simulink model "MSDRPrimaryLoop_LoadFollow"  (R2021b)
settings: Solver=VariableStepAuto  StartTime=0.0  StopTime=604900  MaxStep=1  MinStep=0.01  RelTol=1e-3
undefined symbols (not defined in the file): a_f, A_free_PHX, a_g, A_h_PHX, beta, beta_t, bubbleGeneratorArea, bubbleGeneratorDh, bubbleGeneratorElevation, bubbleGeneratorLength, bubbleGeneratorVolume, bubbleSaturationLevel, bubbleSeparatorArea, bubbleSeparatorDiameter, bubbleSeparatorDo, bubbleSeparatorLength, bubbleSeparatorSlope, bypassRatio, C0, coreFlowArea, coreFuelVolume, coreLowerPlenumArea, coreLowerPlenumHydraulicDiameter, coreLowerPlenumLength, coreLowerPlenumVolume, coreUpperPlenumArea, coreUpperPlenumHydraulicDiameter, coreUpperPlenumLength, coreUpperPlenumVolume, coreVolume, cpGraphite, dissolusionRatio, dMin, dScale, dsmConst, DXeG, Fiss_factor, fuelChannelHydrualicDiameter, fuelChannelLength, fuelDepositRatio, fuelFraction, fuelGraphiteArea, fuelGraphiteHeatTransferCoefficient, gamma0, gamma1, gamma2, generatorDsm, graphiteKDiff, graphiteUnitCellThickness, initialIodineConcentration, InitialXeMolarConcentration, InjectionRatio, injectionRatio, iodineDecayConstant, IodineDecayConstant, iodineYield, kGraphite, kScale, Lam, lam ... (+60)
libraries: fl_lib x268, nesl_utility x106, SimscapeFluids_lib x20, slpidlib x1
(part 10 of 12)

== system MSDRPrimaryLoop_LoadFollow/Chemical Processing/PipeLine/XenonCalc/InterphaseTranfser/Constitutive ==
  alpha : Inport
  PLoss : Inport  Port=2
  VolumeRate : Inport  Port=3
  Diam : Inport  Port=4
  Absolute Reference (TL) : fl_lib/Thermal Liquid/Elements/Absolute Reference (TL)
      settings: SourceProductBaseCode=SS
  DiffusivityScale : Subsystem  ReferencedSubsystem=DiffusivityScale
  Divide : Product  Inputs=**/
  Divide1 : Product  Inputs=*/
  KScale : Subsystem  ReferencedSubsystem=KScale
  PS-Simulink Converter : nesl_utility/PS-Simulink Converter  PhysicalDomain=network_engine_domain  SubClassName=ps_output  LeftPortType=input  RightPortType=output  PseudoPeriodic=off  Frequencies=[]  Unit=inherit  AffineConversion=off
      settings: SourceProductBaseCode=PW,SS
  PS-Simulink Converter2 : nesl_utility/PS-Simulink Converter  PhysicalDomain=network_engine_domain  SubClassName=ps_output  LeftPortType=input  RightPortType=output  PseudoPeriodic=off  Frequencies=[]  Unit=inherit  AffineConversion=off
      settings: SourceProductBaseCode=PW,SS
  Pressure & Temperature Sensor (TL) : fl_lib/Thermal Liquid/Sensors/Pressure & Temperature Sensor (TL)
      settings: SourceProductBaseCode=SS  InternalSimscapePortConfiguration="{\"Bottom\":[],\"Left\":[{\"id\":\"A\",\"label\":\"A\",\"type\":\"foundation.thermal_liquid.thermal_liquid\"}],\"Right\":[{\"id\":\"B\",\"label\":\"B\",\"type\":\"foundation.thermal_liquid.thermal_liquid\"},{\"id\":\"P\",\"label\":\"P\",\"type\":\"output\"},{\"id\":\"T\",\"label\":\"T\",\"type\":\"output\"}],\"Top\":[]}"
  RateToVelocity : Gain  Gain=1/Area
  Simscape Component : SimscapeComponentBlock  SourceFile=TL_FullSensor  ComponentPath=TL_FullSensor  ComponentVariants="[\"TL_FullSensor\"]"  ComponentVariantNames="[\"TL_FullSensor\"]"  ClassName=TL_FullSensor  SchemaVersion=1
      settings: CopyFcn=simscape.engine.sli.internal.componentblockcallback(gcbh,'COPY')  PreCopyFcn=simscape.engine.sli.internal.componentblockcallback(gcbh,'PRECOPY')  PreDeleteFcn=simscape.engine.sli.internal.componentblockcallback(gcbh,'PREDELETE')  InternalSimscapePortConfiguration="{\"Bottom\":[],\"Left\":[{\"id\":\"A\",\"label\":\"A\",\"type\":\"foundation.thermal_liquid.thermal_liquid\"}],\"Right\":[{\"id\":\"U\",\"label\":\"u\",\"type\":\"output\"},{\"id\":\"RHO\",\"label\":\"rho\",\"type\":\"output\"},{\"id\":\"CP\",\"label\":\"cp\",\"type\":\"output\"},{\"id\":\"NU\",\"label\":\"nu\",\"type\":\"output\"}],\"Top\":[]}"
      mask Type: Thermodynamic Properties Sensor (TL)
  Subsystem : Subsystem
      settings: PortSchema="{\"entries\":[{\"content\":{\"sides\":[{\"content\":{\"connectorIds\":[\"In1\",\"In2\",\"In3\"]},\"type\":\"ConnectorPlacement.EquallySpacedRectSide\",\"uuid\":\"dd1c86c2-327e-41b5-90e0-a07cc4f7a239\"},{\"content\":{\"connectorIds\":[\"Out1\",\"Out2\"],\"side\":\"RIGHT\"},\"type\":\"ConnectorPlacement.EquallySpacedRectSide\",\"uuid\":\"1daff71e-8b5d-4f35-9ce7-352085350762\"},{\"content\":{\"connectorIds\":[],\"side\":\"TOP\"},\"type\":\"ConnectorPlacement.EquallySpacedRectSide\",\"uuid\":\"6cf7e847-c1ca-4561-96b9-90e4339d236b\"},{\"content\":{\"connectorIds\":[\"RConn1\"],\"side\":\"BOTTOM\"},\"type\":\"ConnectorPlacement.EquallySpacedRectSide\",\"uuid\":\"444ecab7-0e05-438f-8395-0556f9cb1910\"}]},\"type\":\"ConnectorPlacement.EquallySpacedConnector\",\"uuid\":\"a820de5e-57ef-4a78-919f-756fbb4a48db\"}],\"packageUris\":[\"http://schema.mathworks.com/mf0/Connector/R2020b\"],\"version\":\"1.0\"}"
  Ref : PMIOPort  Side=Left
  ul : Outport
  ug : Outport  Port=2
  K : Outport  Port=3
  Re : Outport  Port=4
  Sc : Outport  Port=5
  Diff : Outport  Port=6
  alphaC : Outport  Port=7
  dsm : Outport  Port=8
  f_m : Outport  Port=9
  wires:
  alpha/1 -> alphaC/1
  VolumeRate/1 -> RateToVelocity/1
  RateToVelocity/1 -> ug/1, Subsystem/3(ul), ul/1, Divide/1
  Diam/1 -> Subsystem/2(Dh), Divide/2
  PS-Simulink Converter/1 -> Divide/3, Divide1/1
  PS-Simulink Converter2/1 -> DiffusivityScale/1, KScale/1
  DiffusivityScale/1 -> Divide1/2, Diff/1
  Divide1/1 -> Sc/1
  KScale/1 -> K/1
  Subsystem/2(dsm) -> dsm/1
  Divide/1 -> Re/1
  Subsystem/1(f_Combined) -> f_m/1
  PLoss/1 -> Subsystem/1(PLoss)
  connections:
  Pressure & Temperature Sensor (TL)/LConn1 -- Simscape Component/LConn1 -- Ref/RConn1 -- Subsystem/RConn1
  Simscape Component/RConn4 -- PS-Simulink Converter/LConn1
  Pressure & Temperature Sensor (TL)/RConn3 -- PS-Simulink Converter2/LConn1
  Pressure & Temperature Sensor (TL)/RConn1 -- Absolute Reference (TL)/LConn1

== system MSDRPrimaryLoop_LoadFollow/Chemical Processing/PipeLine/XenonCalc/Salt/InPipeGeneration ==
  IodineSNumberDensity : Inport
  T_f_ave : Inport  Port=2
  DecayXenonGenerationRate : Product
  Molar/s : Product  Inputs=*/
  Na : Constant  Value=6.022e23
  T2Rho : Fcn  Expr=3960 - 0.6724*u
  gain : Gain  Gain=iodineDecayConstant*Volume
  kg/s : Gain  Gain=0.135
  "XenonGenerationRate, [kg/s]" : Outport
  wires:
  IodineSNumberDensity/1 -> gain/1
  T_f_ave/1 -> T2Rho/1
  gain/1 -> DecayXenonGenerationRate/1
  T2Rho/1 -> DecayXenonGenerationRate/2
  DecayXenonGenerationRate/1 -> Molar/s/1
  Na/1 -> Molar/s/2
  Molar/s/1 -> kg/s/1
  kg/s/1 -> "XenonGenerationRate, [kg/s]"/1

== system MSDRPrimaryLoop_LoadFollow/Chemical Processing/PipeLine/XenonCalc/Salt/Subsystem1 ==
  Gas : Inport
  Add1 : Sum  Inputs=+-
  Constant : Constant
  Subsystem : Subsystem  ReferencedSubsystem=GasToAlpha
  1-alpha : Outport
  wires:
  Gas/1 -> Subsystem/1
  Constant/1 -> Add1/1
  Subsystem/1 -> Add1/2
  Add1/1 -> 1-alpha/1

== system MSDRPrimaryLoop_LoadFollow/PHX/PHX Ideal/XenonCalc/InterphaseTranfser/Constitutive ==
  alpha : Inport
  PLoss : Inport  Port=2
  VolumeRate : Inport  Port=3
  Diam : Inport  Port=4
  Absolute Reference (TL) : fl_lib/Thermal Liquid/Elements/Absolute Reference (TL)
      settings: SourceProductBaseCode=SS
  DiffusivityScale : Subsystem  ReferencedSubsystem=DiffusivityScale
  Divide : Product  Inputs=**/
  Divide1 : Product  Inputs=*/
  KScale : Subsystem  ReferencedSubsystem=KScale
  PS-Simulink Converter : nesl_utility/PS-Simulink Converter  PhysicalDomain=network_engine_domain  SubClassName=ps_output  LeftPortType=input  RightPortType=output  PseudoPeriodic=off  Frequencies=[]  Unit=inherit  AffineConversion=off
      settings: SourceProductBaseCode=PW,SS
  PS-Simulink Converter2 : nesl_utility/PS-Simulink Converter  PhysicalDomain=network_engine_domain  SubClassName=ps_output  LeftPortType=input  RightPortType=output  PseudoPeriodic=off  Frequencies=[]  Unit=inherit  AffineConversion=off
      settings: SourceProductBaseCode=PW,SS
  Pressure & Temperature Sensor (TL) : fl_lib/Thermal Liquid/Sensors/Pressure & Temperature Sensor (TL)
      settings: SourceProductBaseCode=SS  InternalSimscapePortConfiguration="{\"Bottom\":[],\"Left\":[{\"id\":\"A\",\"label\":\"A\",\"type\":\"foundation.thermal_liquid.thermal_liquid\"}],\"Right\":[{\"id\":\"B\",\"label\":\"B\",\"type\":\"foundation.thermal_liquid.thermal_liquid\"},{\"id\":\"P\",\"label\":\"P\",\"type\":\"output\"},{\"id\":\"T\",\"label\":\"T\",\"type\":\"output\"}],\"Top\":[]}"
  RateToVelocity : Gain  Gain=1/Area
  Simscape Component : SimscapeComponentBlock  SourceFile=TL_FullSensor  ComponentPath=TL_FullSensor  ComponentVariants="[\"TL_FullSensor\"]"  ComponentVariantNames="[\"TL_FullSensor\"]"  ClassName=TL_FullSensor  SchemaVersion=1
      settings: CopyFcn=simscape.engine.sli.internal.componentblockcallback(gcbh,'COPY')  PreCopyFcn=simscape.engine.sli.internal.componentblockcallback(gcbh,'PRECOPY')  PreDeleteFcn=simscape.engine.sli.internal.componentblockcallback(gcbh,'PREDELETE')  InternalSimscapePortConfiguration="{\"Bottom\":[],\"Left\":[{\"id\":\"A\",\"label\":\"A\",\"type\":\"foundation.thermal_liquid.thermal_liquid\"}],\"Right\":[{\"id\":\"U\",\"label\":\"u\",\"type\":\"output\"},{\"id\":\"RHO\",\"label\":\"rho\",\"type\":\"output\"},{\"id\":\"CP\",\"label\":\"cp\",\"type\":\"output\"},{\"id\":\"NU\",\"label\":\"nu\",\"type\":\"output\"}],\"Top\":[]}"
      mask Type: Thermodynamic Properties Sensor (TL)
  dsmFun : Subsystem  ReferencedSubsystem=dsmFun
      settings: PortSchema="{\"entries\":[{\"content\":{\"sides\":[{\"content\":{\"connectorIds\":[\"In2\",\"In3\",\"In4\"]},\"type\":\"ConnectorPlacement.EquallySpacedRectSide\",\"uuid\":\"cd878d6d-d881-48a3-8bcf-2f6377bc2619\"},{\"content\":{\"connectorIds\":[\"Out1\",\"Out2\"],\"side\":\"RIGHT\"},\"type\":\"ConnectorPlacement.EquallySpacedRectSide\",\"uuid\":\"84ec48cd-6af4-419c-aaeb-7134212c3ae2\"},{\"content\":{\"connectorIds\":[\"In1\"],\"side\":\"TOP\"},\"type\":\"ConnectorPlacement.EquallySpacedRectSide\",\"uuid\":\"d836bcb8-c56c-40d6-b9ba-0790b759147b\"},{\"content\":{\"connectorIds\":[\"RConn1\"],\"side\":\"BOTTOM\"},\"type\":\"ConnectorPlacement.EquallySpacedRectSide\",\"uuid\":\"16763d39-53e3-4dc4-9c8a-2531c5df2d8d\"}]},\"type\":\"ConnectorPlacement.EquallySpacedConnector\",\"uuid\":\"ad3a93fd-9624-45a3-bd6b-21e42fcd018d\"}],\"packageUris\":[\"http://schema.mathworks.com/mf0/Connector/R2020b\"],\"version\":\"1.0\"}"
  Ref : PMIOPort  Side=Left
  ul : Outport
  ug : Outport  Port=2
  K : Outport  Port=3
  Re : Outport  Port=4
  Sc : Outport  Port=5
  Diff : Outport  Port=6
  alphaC : Outport  Port=7
  dsm : Outport  Port=8
  f_m : Outport  Port=9
  wires:
  alpha/1 -> alphaC/1, dsmFun/1
  VolumeRate/1 -> RateToVelocity/1
  RateToVelocity/1 -> ug/1, dsmFun/4, ul/1, Divide/1
  Diam/1 -> Divide/2, dsmFun/3
  PS-Simulink Converter/1 -> Divide/3, Divide1/1
  PS-Simulink Converter2/1 -> DiffusivityScale/1, KScale/1
  DiffusivityScale/1 -> Divide1/2, Diff/1
  Divide1/1 -> Sc/1
  KScale/1 -> K/1
  dsmFun/2 -> dsm/1
  Divide/1 -> Re/1
  dsmFun/1 -> f_m/1
  PLoss/1 -> dsmFun/2
  connections:
  Pressure & Temperature Sensor (TL)/LConn1 -- dsmFun/RConn1 -- Simscape Component/LConn1 -- Ref/RConn1
  Simscape Component/RConn4 -- PS-Simulink Converter/LConn1
  Pressure & Temperature Sensor (TL)/RConn3 -- PS-Simulink Converter2/LConn1
  Pressure & Temperature Sensor (TL)/RConn1 -- Absolute Reference (TL)/LConn1

== system MSDRPrimaryLoop_LoadFollow/PHX/PHX Ideal/XenonCalc/Salt/InPipeGeneration ==
  IodineSNumberDensity : Inport
  T_f_ave : Inport  Port=2
  DecayXenonGenerationRate : Product
  Molar/s : Product  Inputs=*/
  Na : Constant  Value=6.022e23
  T2Rho : Fcn  Expr=3960 - 0.6724*u
  gain : Gain  Gain=iodineDecayConstant*Volume
  kg/s : Gain  Gain=0.135
  "XenonGenerationRate, [kg/s]" : Outport
  wires:
  IodineSNumberDensity/1 -> gain/1
  T_f_ave/1 -> T2Rho/1
  gain/1 -> DecayXenonGenerationRate/1
  T2Rho/1 -> DecayXenonGenerationRate/2
  DecayXenonGenerationRate/1 -> Molar/s/1
  Na/1 -> Molar/s/2
  Molar/s/1 -> kg/s/1
  kg/s/1 -> "XenonGenerationRate, [kg/s]"/1

== system MSDRPrimaryLoop_LoadFollow/PHX/PHX Ideal/XenonCalc/Salt/Subsystem1 ==
  Gas : Inport
  Add1 : Sum  Inputs=+-
  Constant : Constant
  Subsystem : Subsystem  ReferencedSubsystem=GasToAlpha
  1-alpha : Outport
  wires:
  Gas/1 -> Subsystem/1
  Constant/1 -> Add1/1
  Subsystem/1 -> Add1/2
  Add1/1 -> 1-alpha/1

== system MSDRPrimaryLoop_LoadFollow/PHX/PHX Physical/XenonCalc1/InterphaseTranfser/Constitutive ==
  alpha : Inport
  VolumeRate : Inport  Port=2
  Diam : Inport  Port=3
  Absolute Reference (TL) : fl_lib/Thermal Liquid/Elements/Absolute Reference (TL)
      settings: SourceProductBaseCode=SS
  DiffusivityScale : Subsystem  ReferencedSubsystem=DiffusivityScale
  Divide : Product  Inputs=**/
  Divide1 : Product  Inputs=*/
  KScale : Subsystem  ReferencedSubsystem=KScale
  PS-Simulink Converter : nesl_utility/PS-Simulink Converter  PhysicalDomain=network_engine_domain  SubClassName=ps_output  LeftPortType=input  RightPortType=output  PseudoPeriodic=off  Frequencies=[]  Unit=inherit  AffineConversion=off
      settings: SourceProductBaseCode=PW,SS
  PS-Simulink Converter1 : nesl_utility/PS-Simulink Converter  PhysicalDomain=network_engine_domain  SubClassName=ps_output  LeftPortType=input  RightPortType=output  PseudoPeriodic=off  Frequencies=[]  Unit=inherit  AffineConversion=off
      settings: SourceProductBaseCode=PW,SS
  PS-Simulink Converter2 : nesl_utility/PS-Simulink Converter  PhysicalDomain=network_engine_domain  SubClassName=ps_output  LeftPortType=input  RightPortType=output  PseudoPeriodic=off  Frequencies=[]  Unit=inherit  AffineConversion=off
      settings: SourceProductBaseCode=PW,SS
  Pressure & Temperature Sensor (TL) : fl_lib/Thermal Liquid/Sensors/Pressure & Temperature Sensor (TL)
      settings: SourceProductBaseCode=SS  InternalSimscapePortConfiguration="{\"Bottom\":[],\"Left\":[{\"id\":\"A\",\"label\":\"A\",\"type\":\"foundation.thermal_liquid.thermal_liquid\"}],\"Right\":[{\"id\":\"B\",\"label\":\"B\",\"type\":\"foundation.thermal_liquid.thermal_liquid\"},{\"id\":\"P\",\"label\":\"P\",\"type\":\"output\"},{\"id\":\"T\",\"label\":\"T\",\"type\":\"output\"}],\"Top\":[]}"
  RateToVelocity : Gain  Gain=1/PipeArea
  Simscape Component : SimscapeComponentBlock  SourceFile=TL_FullSensor  ComponentPath=TL_FullSensor  ComponentVariants="[\"TL_FullSensor\"]"  ComponentVariantNames="[\"TL_FullSensor\"]"  ClassName=TL_FullSensor  SchemaVersion=1
      settings: CopyFcn=simscape.engine.sli.internal.componentblockcallback(gcbh,'COPY')  PreCopyFcn=simscape.engine.sli.internal.componentblockcallback(gcbh,'PRECOPY')  PreDeleteFcn=simscape.engine.sli.internal.componentblockcallback(gcbh,'PREDELETE')  InternalSimscapePortConfiguration="{\"Bottom\":[],\"Left\":[{\"id\":\"A\",\"label\":\"A\",\"type\":\"foundation.thermal_liquid.thermal_liquid\"}],\"Right\":[{\"id\":\"U\",\"label\":\"u\",\"type\":\"output\"},{\"id\":\"RHO\",\"label\":\"rho\",\"type\":\"output\"},{\"id\":\"CP\",\"label\":\"cp\",\"type\":\"output\"},{\"id\":\"NU\",\"label\":\"nu\",\"type\":\"output\"}],\"Top\":[]}"
      mask Type: Thermodynamic Properties Sensor (TL)
  dsmFun : Subsystem  ReferencedSubsystem=dsmFun
      settings: PortSchema="{\"entries\":[{\"content\":{\"sides\":[{\"content\":{\"connectorIds\":[\"In1\",\"In2\",\"In3\",\"In4\"]},\"type\":\"ConnectorPlacement.EquallySpacedRectSide\",\"uuid\":\"cd878d6d-d881-48a3-8bcf-2f6377bc2619\"},{\"content\":{\"connectorIds\":[\"Out1\",\"Out2\"],\"side\":\"RIGHT\"},\"type\":\"ConnectorPlacement.EquallySpacedRectSide\",\"uuid\":\"84ec48cd-6af4-419c-aaeb-7134212c3ae2\"},{\"content\":{\"connectorIds\":[],\"side\":\"TOP\"},\"type\":\"ConnectorPlacement.EquallySpacedRectSide\",\"uuid\":\"d836bcb8-c56c-40d6-b9ba-0790b759147b\"},{\"content\":{\"connectorIds\":[\"RConn1\"],\"side\":\"BOTTOM\"},\"type\":\"ConnectorPlacement.EquallySpacedRectSide\",\"uuid\":\"16763d39-53e3-4dc4-9c8a-2531c5df2d8d\"}]},\"type\":\"ConnectorPlacement.EquallySpacedConnector\",\"uuid\":\"ad3a93fd-9624-45a3-bd6b-21e42fcd018d\"}],\"packageUris\":[\"http://schema.mathworks.com/mf0/Connector/R2020b\"],\"version\":\"1.0\"}"
  Ref : PMIOPort  Side=Left
  ul : Outport
  ug : Outport  Port=2
  K : Outport  Port=3
  Re : Outport  Port=4
  Sc : Outport  Port=5
  Diff : Outport  Port=6
  alphaC : Outport  Port=7
  dsm : Outport  Port=8
  wires:
  alpha/1 -> alphaC/1
  VolumeRate/1 -> RateToVelocity/1
  RateToVelocity/1 -> ug/1, dsmFun/3, ul/1, Divide/1
  Diam/1 -> dsmFun/2, Divide/2
  PS-Simulink Converter/1 -> Divide/3, Divide1/1
  PS-Simulink Converter1/1 -> DiffusivityScale/1
  PS-Simulink Converter2/1 -> KScale/1
  DiffusivityScale/1 -> Divide1/2, Diff/1
  Divide1/1 -> Sc/1
  KScale/1 -> K/1
  dsmFun/1 -> dsm/1
  Divide/1 -> dsmFun/1, Re/1
  connections:
  Pressure & Temperature Sensor (TL)/LConn1 -- dsmFun/RConn1 -- Simscape Component/LConn1 -- Ref/RConn1
  Simscape Component/RConn4 -- PS-Simulink Converter/LConn1
  Simscape Component/RConn2 -- PS-Simulink Converter1/LConn1
  Pressure & Temperature Sensor (TL)/RConn3 -- PS-Simulink Converter2/LConn1
  Pressure & Temperature Sensor (TL)/RConn1 -- Absolute Reference (TL)/LConn1

== system MSDRPrimaryLoop_LoadFollow/PHX/PHX Physical/XenonCalc1/Salt/InPipeGeneration ==
  IodineSNumberDensity : Inport
  T_f_ave : Inport  Port=2
  DecayXenonGenerationRate : Product
  Molar/s : Product  Inputs=*/
  Na : Constant  Value=6.022e23
  T2Rho : Fcn  Expr=3.9603e+03 - 0.6724*u
  gain : Gain  Gain=IodineDecayConstant*PipeVolume
  kg/s : Gain  Gain=0.135
  "XenonGenerationRate, [kg/s]" : Outport
  wires:
  IodineSNumberDensity/1 -> gain/1
  T_f_ave/1 -> T2Rho/1
  gain/1 -> DecayXenonGenerationRate/1
  T2Rho/1 -> DecayXenonGenerationRate/2
  DecayXenonGenerationRate/1 -> Molar/s/1
  Na/1 -> Molar/s/2
  Molar/s/1 -> kg/s/1
  kg/s/1 -> "XenonGenerationRate, [kg/s]"/1

== system MSDRPrimaryLoop_LoadFollow/PHX/PHX Physical/XenonCalc1/Salt/Subsystem1 ==
  Gas : Inport
  Add1 : Sum  Inputs=+-
  Constant : Constant
  Subsystem : Subsystem  ReferencedSubsystem=GasToAlpha
  1-alpha : Outport
  wires:
  Gas/1 -> Subsystem/1
  Constant/1 -> Add1/1
  Subsystem/1 -> Add1/2
  Add1/1 -> 1-alpha/1

== system MSDRPrimaryLoop_LoadFollow/Pump/PumpIdeal/XenonCalcPump/InterphaseTranfser/Constitutive ==
  Absolute Reference (TL) : fl_lib/Thermal Liquid/Elements/Absolute Reference (TL)
      settings: SourceProductBaseCode=SS
  Constant : Constant  Value=dsm
  Constant1 : Constant  Value=km
  KScale : Subsystem  ReferencedSubsystem=KScale
  PS-Simulink Converter2 : nesl_utility/PS-Simulink Converter  PhysicalDomain=network_engine_domain  SubClassName=ps_output  LeftPortType=input  RightPortType=output  PseudoPeriodic=off  Frequencies=[]  Unit=inherit  AffineConversion=off
      settings: SourceProductBaseCode=PW,SS
  Pressure & Temperature Sensor (TL) : fl_lib/Thermal Liquid/Sensors/Pressure & Temperature Sensor (TL)
      settings: SourceProductBaseCode=SS  InternalSimscapePortConfiguration="{\"Bottom\":[],\"Left\":[{\"id\":\"A\",\"label\":\"A\",\"type\":\"foundation.thermal_liquid.thermal_liquid\"}],\"Right\":[{\"id\":\"B\",\"label\":\"B\",\"type\":\"foundation.thermal_liquid.thermal_liquid\"},{\"id\":\"P\",\"label\":\"P\",\"type\":\"output\"},{\"id\":\"T\",\"label\":\"T\",\"type\":\"output\"}],\"Top\":[]}"
  Ref : PMIOPort  Side=Left
  K : Outport
  dsm : Outport  Port=2
  k : Outport  Port=3
  wires:
  PS-Simulink Converter2/1 -> KScale/1
  KScale/1 -> K/1
  Constant/1 -> dsm/1
  Constant1/1 -> k/1
  connections:
  Pressure & Temperature Sensor (TL)/LConn1 -- Ref/RConn1
  Pressure & Temperature Sensor (TL)/RConn3 -- PS-Simulink Converter2/LConn1
  Pressure & Temperature Sensor (TL)/RConn1 -- Absolute Reference (TL)/LConn1

== system MSDRPrimaryLoop_LoadFollow/Pump/PumpIdeal/XenonCalcPump/Salt/InPipeGeneration ==
  IodineSNumberDensity : Inport
  T_f_ave : Inport  Port=2
  DecayXenonGenerationRate : Product
  Molar/s : Product  Inputs=*/
  Na : Constant  Value=6.022e23
  T2Rho : Fcn  Expr=3960 - 0.6724*u
  gain : Gain  Gain=iodineDecayConstant*PipeVolume
  kg/s : Gain  Gain=0.135
  "XenonGenerationRate, [kg/s]" : Outport
  wires:
  IodineSNumberDensity/1 -> gain/1
  T_f_ave/1 -> T2Rho/1
  gain/1 -> DecayXenonGenerationRate/1
  T2Rho/1 -> DecayXenonGenerationRate/2
  DecayXenonGenerationRate/1 -> Molar/s/1
  Na/1 -> Molar/s/2
  Molar/s/1 -> kg/s/1
  kg/s/1 -> "XenonGenerationRate, [kg/s]"/1

== system MSDRPrimaryLoop_LoadFollow/Pump/PumpIdeal/XenonCalcPump/Salt/Subsystem1 ==
  Gas : Inport
  Add1 : Sum  Inputs=+-
  Constant : Constant
  Subsystem : Subsystem  ReferencedSubsystem=GasToAlpha
  1-alpha : Outport
  wires:
  Gas/1 -> Subsystem/1
  Constant/1 -> Add1/1
  Subsystem/1 -> Add1/2
  Add1/1 -> 1-alpha/1

== system MSDRPrimaryLoop_LoadFollow/Reactor/CoreTH&Inerti/Core/CoreTH/CoreLinearNode ==
  note: Private model diameters are for MSDR only. These are based on the slab geometry and are not applicable to different reactor core design.
  note: Model with 1D simplified cylindrical quasi static heat transfer. Bi=0.26.
      | Refer to Nuclear Systems: 8.5.6. Or FHMT:5.5.2.
      | This is roughly ok for lumped analysis.
  GasRef : Inport
  2PModification : Subsystem  ReferencedSubsystem=TwoPhaseModification
      settings: PortSchema="{\"entries\":[{\"content\":{\"sides\":[{\"content\":{\"connectorIds\":[\"LConn1\"]},\"type\":\"ConnectorPlacement.EquallySpacedRectSide\",\"uuid\":\"7546b4b7-b669-49c8-8f27-f696391ea3ad\"},{\"content\":{\"connectorIds\":[\"RConn1\"],\"side\":\"RIGHT\"},\"type\":\"ConnectorPlacement.EquallySpacedRectSide\",\"uuid\":\"0e6176f2-177c-4327-bcfa-9a190fe9083f\"},{\"content\":{\"connectorIds\":[\"LConn2\",\"In1\"],\"side\":\"TOP\"},\"type\":\"ConnectorPlacement.EquallySpacedRectSide\",\"uuid\":\"16faf74c-4635-4009-a5b3-33dd03b625c6\"},{\"content\":{\"connectorIds\":[\"RConn2\"],\"side\":\"BOTTOM\"},\"type\":\"ConnectorPlacement.EquallySpacedRectSide\",\"uuid\":\"2081d73b-bb08-4ad9-b5c8-e48a4e9c4e20\"}]},\"type\":\"ConnectorPlacement.EquallySpacedConnector\",\"uuid\":\"243e4075-206b-4747-a8bc-b8f10d9a577f\"}],\"packageUris\":[\"http://schema.mathworks.com/mf0/Connector/R2020b\"],\"version\":\"1.0\"}"
  Conductive Heat Transfer1 : fl_lib/Thermal/Thermal Elements/Conductive Heat Transfer  area=CoreVolume/CoreLength*(1-FuelFraction) m^2  thickness=0.5*CoreLength/N_nodes m  th_cond=k_graphite W/(m*K)  T_specify=off  T_priority=None  T=0 K  T_nominal_specify=off  T_nominal_unit=K  T_nominal_value=1  Q_specify=off  Q_priority=None  Q=0 W  Q_nominal_specify=off  Q_nominal_unit=W  Q_nominal_value=1
  Conductive Heat Transfer2 : fl_lib/Thermal/Thermal Elements/Conductive Heat Transfer  area=CoreVolume/CoreLength*(1-FuelFraction) m^2  thickness=0.5*CoreLength/N_nodes m  th_cond=k_graphite W/(m*K)  T_specify=off  T_priority=None  T=0 K  T_nominal_specify=off  T_nominal_unit=K  T_nominal_value=1  Q_specify=off  Q_priority=None  Q=0 W  Q_nominal_specify=off  Q_nominal_unit=W  Q_nominal_value=1
  Conductive Heat Transfer3 : fl_lib/Thermal/Thermal Elements/Conductive Heat Transfer  area=FuelGraphiteArea/N_nodes m^2  thickness=0.5*UnitCellGraphiteThickness m  th_cond=k_graphite W/(m*K)  T_specify=off  T_priority=None  T=0 K  T_nominal_specify=off  T_nominal_unit=K  T_nominal_value=1  Q_specify=off  Q_priority=None  Q=0 W  Q_nominal_specify=off  Q_nominal_unit=W  Q_nominal_value=1
  Constant Volume Chamber (TL) : fl_lib/Thermal Liquid/Elements/Constant Volume Chamber (TL)  volume=0.001 m^3  num_ports=foundation.enum.num_ports.two  area_A=0.01 m^2  area_B=0.01 m^2  area_C=0.01 m^2  area_D=0.01 m^2  p_I_specify=on  p_I_priority=None  p_I=P0 Pa  p_I_nominal_specify=off  p_I_nominal_unit=MPa  p_I_nominal_value=1  T_I_specify=on  T_I_priority=None  T_I=T0 K  T_I_nominal_specify=off  T_I_nominal_unit=K  T_I_nominal_value=1  u_chamber_specify=on  u_chamber_priority=None  u_chamber=cpMSRE J/kg  u_chamber_nominal_specify=off  u_chamber_nominal_unit=kJ/kg  u_chamber_nominal_value=1  rho_specify=on  rho_priority=None  rho=nominalFuelDensity kg/m^3  rho_nominal_specify=off  rho_nominal_unit=kg/m^3  rho_nominal_value=1
      settings: SourceProductBaseCode=SS  LogSimulationData=on  InternalSimscapePortConfiguration="{\"Bottom\":[],\"Left\":[{\"id\":\"A\",\"label\":\"A\",\"type\":\"foundation.thermal_liquid.thermal_liquid\"},{\"id\":\"H\",\"label\":\"H\",\"type\":\"foundation.thermal.thermal\"}],\"Right\":[{\"id\":\"B\",\"label\":\"B\",\"type\":\"foundation.thermal_liquid.thermal_liquid\"}],\"Top\":[]}"
  Controlled Heat Flow Rate Source : fl_lib/Thermal/Thermal Sources/Controlled Heat Flow Rate Source
      settings: LogSimulationData=on
  Convective Heat Transfer : fl_lib/Thermal/Thermal Elements/Convective Heat Transfer  area=fuelGraphiteArea/N_nodes m^2  heat_tr_coeff=fuelGraphiteHeatTransferCoefficient W/(m^2*K)  T_specify=off  T_priority=None  T=0 K  T_nominal_specify=off  T_nominal_unit=K  T_nominal_value=1  Q_specify=off  Q_priority=None  Q=0 W  Q_nominal_specify=off  Q_nominal_unit=W  Q_nominal_value=1
  Fuel Deposited : fl_lib/Physical Signals/Functions/PS Gain  gain=FuelDepositRatio*CoreVolume/N_nodes m^3
  Grahite Deposited : fl_lib/Thermal/Thermal Sources/Controlled Heat Flow Rate Source
      settings: LogSimulationData=on
  Graphite Deposited : fl_lib/Physical Signals/Functions/PS Gain  gain=(1-FuelDepositRatio)*CoreVolume/N_nodes m^3
  Pipe (TL) : SimscapeFluids_lib/Thermal Liquid/Pipes & Fittings/Pipe (TL)  dynamic_compressibility=simscape.enum.onoff.on  inertia=simscape.enum.onoff.off  num_segments=1  pipe_length=fuelChannelLength/N_nodes m  area=coreFlowArea m^2  Dh=0.1128 m  wall_spec=fluids.thermal_liquid.pipes_fittings.enum.wall_spec.rigid  Dh_rigid=fuelChannelHydrualicDiameter m  wall_compliance=1.2e-6 m/MPa  wall_time_constant=0.01 s  elevation_spec=foundation.enum.constant_variable.constant  elevation_gain=fuelChannelLength/N_nodes m  g=9.82 m/s^2  pressure_loss_spec=fluids.thermal_liquid.pipes_fittings.enum.PressureLossSpec.Haaland  length_add=1 m  roughness=surfaceRoughness m  Re_friction_TLU=[400, 1000, 1500, 3000, 4000, 6000, 10000, 20000, 40000, 60000, 100000, 100000000]  friction_factor_TLU=[.264, .112, .071, .0417, .0387, .0268, .025, .0232, .0226, .022, .0214, .0214]  shape_factor=64  Re_lam=2000  Re_tur=4000  mdot_nominal=[.1, 1] kg/s  p_diff_nominal=[.001, .01] MPa  mdot_threshold=1e-6 kg/s  heat_transfer_spec=fluids.thermal_liquid.pipes_fittings.enum.HeatTransferSpec.Gnielinski  mdot_nominal_heat=[0.1, 10000] kg/s  T_in_nominal=[T0, T0] K  T_out_nominal=[T0, T0] K  p_in_nominal_heat=[.101325, .101325] MPa  T_wall_nominal=[T0+1, T0+1] K  a_coeff=0.023  b_Re_power=0.8  c_Pr_power=0.4  Nu_lam=3.66  Re_Colburn_TLU=[100, 150, 1000]  Colburn_factor_TLU=[.019, .013, .002]  Re_Nu_TLU=[100, 150, 1000]  Pr_Nu_TLU=[1, 10]  Nu_TLU=[3.72, 4.21; 3.75, 4.44; 4.21, 7.15]  T0_vec=T0 K  p0_vec=P0 Pa  mdot0=0.1 kg/s
      settings: SourceProductBaseCode=SH
  Temperature Sensor : fl_lib/Thermal/Thermal Sensors/Temperature Sensor
  Thermal Mass : fl_lib/Thermal/Thermal Elements/Thermal Mass  mass=CoreVolume*(1-FuelFraction)*rho_graphite/N_nodes kg  sp_heat=cp_graphite J/(K*kg)  T_specify=on  T_priority=High  T=T0 K  T_nominal_specify=off  T_nominal_unit=K  T_nominal_value=1  Q_specify=off  Q_priority=None  Q=0 W  Q_nominal_specify=off  Q_nominal_unit=W  Q_nominal_value=1
      settings: LogSimulationData=on
  Thermal Reference : fl_lib/Thermal/Thermal Elements/Thermal Reference
  Thermal Reference1 : fl_lib/Thermal/Thermal Elements/Thermal Reference
  Thermal Reference2 : fl_lib/Thermal/Thermal Elements/Thermal Reference
  Inlet : PMIOPort  Side=Left
  GraphiteA : PMIOPort  Port=2  Side=Left
  PowerDensity : PMIOPort  Port=3  Side=Left
  Outlet : PMIOPort  Port=4  Side=Right
  GraphiteB : PMIOPort  Port=5  Side=Right
  FuelTemp : PMIOPort  Port=6  Side=Right
  wires:
  GasRef/1 -> 2PModification/1
  connections:
  Grahite Deposited/LConn1 -- Conductive Heat Transfer3/RConn1 -- Conductive Heat Transfer2/RConn1 -- Thermal Mass/LConn1 -- Conductive Heat Transfer1/LConn1
  Graphite Deposited/LConn1 -- Fuel Deposited/LConn1 -- PowerDensity/RConn1
  Conductive Heat Transfer1/RConn1 -- GraphiteB/RConn1
  Grahite Deposited/RConn1 -- Graphite Deposited/RConn1
  GraphiteA/RConn1 -- Conductive Heat Transfer2/LConn1
  Controlled Heat Flow Rate Source/RConn2 -- Thermal Reference/LConn1
  Grahite Deposited/RConn2 -- Thermal Reference1/LConn1
  Fuel Deposited/RConn1 -- Controlled Heat Flow Rate Source/RConn1
  Outlet/RConn1 -- 2PModification/RConn1
  Temperature Sensor/RConn1 -- Thermal Reference2/LConn1
  Temperature Sensor/RConn2 -- FuelTemp/RConn1
  Inlet/RConn1 -- Constant Volume Chamber (TL)/LConn1
  Temperature Sensor/LConn1 -- Convective Heat Transfer/RConn1 -- Conductive Heat Transfer3/LConn1
  Convective Heat Transfer/LConn1 -- Controlled Heat Flow Rate Source/LConn1 -- Pipe (TL)/LConn2 -- Constant Volume Chamber (TL)/LConn2
  2PModification/LConn1 -- Pipe (TL)/RConn1 -- 2PModification/RConn2
  2PModification/LConn2 -- Pipe (TL)/LConn1 -- Constant Volume Chamber (TL)/RConn1

== system MSDRPrimaryLoop_LoadFollow/Reactor/CoreTH&Inerti/Core/CoreTH/CoreLinearNode1 ==
  note: Private model diameters are for MSDR only. These are based on the slab geometry and are not applicable to different reactor core design.
  note: Model with 1D simplified cylindrical quasi static heat transfer. Bi=0.26.
      | Refer to Nuclear Systems: 8.5.6. Or FHMT:5.5.2.
      | This is roughly ok for lumped analysis.
  GasRef : Inport
  2PModification : Subsystem  ReferencedSubsystem=TwoPhaseModification
      settings: PortSchema="{\"entries\":[{\"content\":{\"sides\":[{\"content\":{\"connectorIds\":[\"LConn1\"]},\"type\":\"ConnectorPlacement.EquallySpacedRectSide\",\"uuid\":\"7546b4b7-b669-49c8-8f27-f696391ea3ad\"},{\"content\":{\"connectorIds\":[\"RConn1\"],\"side\":\"RIGHT\"},\"type\":\"ConnectorPlacement.EquallySpacedRectSide\",\"uuid\":\"0e6176f2-177c-4327-bcfa-9a190fe9083f\"},{\"content\":{\"connectorIds\":[\"LConn2\",\"In1\"],\"side\":\"TOP\"},\"type\":\"ConnectorPlacement.EquallySpacedRectSide\",\"uuid\":\"16faf74c-4635-4009-a5b3-33dd03b625c6\"},{\"content\":{\"connectorIds\":[\"RConn2\"],\"side\":\"BOTTOM\"},\"type\":\"ConnectorPlacement.EquallySpacedRectSide\",\"uuid\":\"2081d73b-bb08-4ad9-b5c8-e48a4e9c4e20\"}]},\"type\":\"ConnectorPlacement.EquallySpacedConnector\",\"uuid\":\"243e4075-206b-4747-a8bc-b8f10d9a577f\"}],\"packageUris\":[\"http://schema.mathworks.com/mf0/Connector/R2020b\"],\"version\":\"1.0\"}"
  Conductive Heat Transfer1 : fl_lib/Thermal/Thermal Elements/Conductive Heat Transfer  area=CoreVolume/CoreLength*(1-FuelFraction) m^2  thickness=0.5*CoreLength/N_nodes m  th_cond=k_graphite W/(m*K)  T_specify=off  T_priority=None  T=0 K  T_nominal_specify=off  T_nominal_unit=K  T_nominal_value=1  Q_specify=off  Q_priority=None  Q=0 W  Q_nominal_specify=off  Q_nominal_unit=W  Q_nominal_value=1
  Conductive Heat Transfer2 : fl_lib/Thermal/Thermal Elements/Conductive Heat Transfer  area=CoreVolume/CoreLength*(1-FuelFraction) m^2  thickness=0.5*CoreLength/N_nodes m  th_cond=k_graphite W/(m*K)  T_specify=off  T_priority=None  T=0 K  T_nominal_specify=off  T_nominal_unit=K  T_nominal_value=1  Q_specify=off  Q_priority=None  Q=0 W  Q_nominal_specify=off  Q_nominal_unit=W  Q_nominal_value=1
  Conductive Heat Transfer3 : fl_lib/Thermal/Thermal Elements/Conductive Heat Transfer  area=FuelGraphiteArea/N_nodes m^2  thickness=0.5*UnitCellGraphiteThickness m  th_cond=k_graphite W/(m*K)  T_specify=off  T_priority=None  T=0 K  T_nominal_specify=off  T_nominal_unit=K  T_nominal_value=1  Q_specify=off  Q_priority=None  Q=0 W  Q_nominal_specify=off  Q_nominal_unit=W  Q_nominal_value=1
  Constant Volume Chamber (TL) : fl_lib/Thermal Liquid/Elements/Constant Volume Chamber (TL)  volume=0.001 m^3  num_ports=foundation.enum.num_ports.two  area_A=0.01 m^2  area_B=0.01 m^2  area_C=0.01 m^2  area_D=0.01 m^2  p_I_specify=on  p_I_priority=None  p_I=P0 Pa  p_I_nominal_specify=off  p_I_nominal_unit=MPa  p_I_nominal_value=1  T_I_specify=on  T_I_priority=None  T_I=T0 K  T_I_nominal_specify=off  T_I_nominal_unit=K  T_I_nominal_value=1  u_chamber_specify=on  u_chamber_priority=None  u_chamber=cpMSRE J/kg  u_chamber_nominal_specify=off  u_chamber_nominal_unit=kJ/kg  u_chamber_nominal_value=1  rho_specify=on  rho_priority=None  rho=nominalFuelDensity kg/m^3  rho_nominal_specify=off  rho_nominal_unit=kg/m^3  rho_nominal_value=1
      settings: SourceProductBaseCode=SS  LogSimulationData=on  InternalSimscapePortConfiguration="{\"Bottom\":[],\"Left\":[{\"id\":\"A\",\"label\":\"A\",\"type\":\"foundation.thermal_liquid.thermal_liquid\"},{\"id\":\"H\",\"label\":\"H\",\"type\":\"foundation.thermal.thermal\"}],\"Right\":[{\"id\":\"B\",\"label\":\"B\",\"type\":\"foundation.thermal_liquid.thermal_liquid\"}],\"Top\":[]}"
  Controlled Heat Flow Rate Source : fl_lib/Thermal/Thermal Sources/Controlled Heat Flow Rate Source
      settings: LogSimulationData=on
  Convective Heat Transfer : fl_lib/Thermal/Thermal Elements/Convective Heat Transfer  area=fuelGraphiteArea/N_nodes m^2  heat_tr_coeff=fuelGraphiteHeatTransferCoefficient W/(m^2*K)  T_specify=off  T_priority=None  T=0 K  T_nominal_specify=off  T_nominal_unit=K  T_nominal_value=1  Q_specify=off  Q_priority=None  Q=0 W  Q_nominal_specify=off  Q_nominal_unit=W  Q_nominal_value=1
  Fuel Deposited : fl_lib/Physical Signals/Functions/PS Gain  gain=FuelDepositRatio*CoreVolume/N_nodes m^3
  Grahite Deposited : fl_lib/Thermal/Thermal Sources/Controlled Heat Flow Rate Source
      settings: LogSimulationData=on
  Graphite Deposited : fl_lib/Physical Signals/Functions/PS Gain  gain=(1-FuelDepositRatio)*CoreVolume/N_nodes m^3
  Pipe (TL) : SimscapeFluids_lib/Thermal Liquid/Pipes & Fittings/Pipe (TL)  dynamic_compressibility=simscape.enum.onoff.on  inertia=simscape.enum.onoff.off  num_segments=1  pipe_length=fuelChannelLength/N_nodes m  area=coreFlowArea m^2  Dh=0.1128 m  wall_spec=fluids.thermal_liquid.pipes_fittings.enum.wall_spec.rigid  Dh_rigid=fuelChannelHydrualicDiameter m  wall_compliance=1.2e-6 m/MPa  wall_time_constant=0.01 s  elevation_spec=foundation.enum.constant_variable.constant  elevation_gain=fuelChannelLength/N_nodes m  g=9.82 m/s^2  pressure_loss_spec=fluids.thermal_liquid.pipes_fittings.enum.PressureLossSpec.Haaland  length_add=1 m  roughness=surfaceRoughness m  Re_friction_TLU=[400, 1000, 1500, 3000, 4000, 6000, 10000, 20000, 40000, 60000, 100000, 100000000]  friction_factor_TLU=[.264, .112, .071, .0417, .0387, .0268, .025, .0232, .0226, .022, .0214, .0214]  shape_factor=64  Re_lam=2000  Re_tur=4000  mdot_nominal=[.1, 1] kg/s  p_diff_nominal=[.001, .01] MPa  mdot_threshold=1e-6 kg/s  heat_transfer_spec=fluids.thermal_liquid.pipes_fittings.enum.HeatTransferSpec.Gnielinski  mdot_nominal_heat=[0.1, 10000] kg/s  T_in_nominal=[T0, T0] K  T_out_nominal=[T0, T0] K  p_in_nominal_heat=[.101325, .101325] MPa  T_wall_nominal=[T0+1, T0+1] K  a_coeff=0.023  b_Re_power=0.8  c_Pr_power=0.4  Nu_lam=3.66  Re_Colburn_TLU=[100, 150, 1000]  Colburn_factor_TLU=[.019, .013, .002]  Re_Nu_TLU=[100, 150, 1000]  Pr_Nu_TLU=[1, 10]  Nu_TLU=[3.72, 4.21; 3.75, 4.44; 4.21, 7.15]  T0_vec=T0 K  p0_vec=P0 Pa  mdot0=0.1 kg/s
      settings: SourceProductBaseCode=SH
  Temperature Sensor : fl_lib/Thermal/Thermal Sensors/Temperature Sensor
  Thermal Mass : fl_lib/Thermal/Thermal Elements/Thermal Mass  mass=CoreVolume*(1-FuelFraction)*rho_graphite/N_nodes kg  sp_heat=cp_graphite J/(K*kg)  T_specify=on  T_priority=High  T=T0 K  T_nominal_specify=off  T_nominal_unit=K  T_nominal_value=1  Q_specify=off  Q_priority=None  Q=0 W  Q_nominal_specify=off  Q_nominal_unit=W  Q_nominal_value=1
      settings: LogSimulationData=on
  Thermal Reference : fl_lib/Thermal/Thermal Elements/Thermal Reference
  Thermal Reference1 : fl_lib/Thermal/Thermal Elements/Thermal Reference
  Thermal Reference2 : fl_lib/Thermal/Thermal Elements/Thermal Reference
  Inlet : PMIOPort  Side=Left
  GraphiteA : PMIOPort  Port=2  Side=Left
  PowerDensity : PMIOPort  Port=3  Side=Left
  Outlet : PMIOPort  Port=4  Side=Right
  GraphiteB : PMIOPort  Port=5  Side=Right
  FuelTemp : PMIOPort  Port=6  Side=Right
  wires:
  GasRef/1 -> 2PModification/1
  connections:
  Grahite Deposited/LConn1 -- Conductive Heat Transfer3/RConn1 -- Conductive Heat Transfer2/RConn1 -- Thermal Mass/LConn1 -- Conductive Heat Transfer1/LConn1
  Graphite Deposited/LConn1 -- Fuel Deposited/LConn1 -- PowerDensity/RConn1
  Conductive Heat Transfer1/RConn1 -- GraphiteB/RConn1
  Grahite Deposited/RConn1 -- Graphite Deposited/RConn1
  GraphiteA/RConn1 -- Conductive Heat Transfer2/LConn1
  Controlled Heat Flow Rate Source/RConn2 -- Thermal Reference/LConn1
  Grahite Deposited/RConn2 -- Thermal Reference1/LConn1
  Fuel Deposited/RConn1 -- Controlled Heat Flow Rate Source/RConn1
  Outlet/RConn1 -- 2PModification/RConn1
  Temperature Sensor/RConn1 -- Thermal Reference2/LConn1
  Temperature Sensor/RConn2 -- FuelTemp/RConn1
  Inlet/RConn1 -- Constant Volume Chamber (TL)/LConn1
  Conductive Heat Transfer3/LConn1 -- Temperature Sensor/LConn1 -- Convective Heat Transfer/RConn1
  Constant Volume Chamber (TL)/LConn2 -- Convective Heat Transfer/LConn1 -- Controlled Heat Flow Rate Source/LConn1 -- Pipe (TL)/LConn2
  2PModification/RConn2 -- 2PModification/LConn1 -- Pipe (TL)/RConn1
  Constant Volume Chamber (TL)/RConn1 -- 2PModification/LConn2 -- Pipe (TL)/LConn1

== system MSDRPrimaryLoop_LoadFollow/Reactor/CoreTH&Inerti/Core/CoreTH/CoreLinearNode2 ==
  note: Private model diameters are for MSDR only. These are based on the slab geometry and are not applicable to different reactor core design.
  note: Model with 1D simplified cylindrical quasi static heat transfer. Bi=0.26.
      | Refer to Nuclear Systems: 8.5.6. Or FHMT:5.5.2.
      | This is roughly ok for lumped analysis.
  GasRef : Inport
  2PModification : Subsystem  ReferencedSubsystem=TwoPhaseModification
      settings: PortSchema="{\"entries\":[{\"content\":{\"sides\":[{\"content\":{\"connectorIds\":[\"LConn1\"]},\"type\":\"ConnectorPlacement.EquallySpacedRectSide\",\"uuid\":\"7546b4b7-b669-49c8-8f27-f696391ea3ad\"},{\"content\":{\"connectorIds\":[\"RConn1\"],\"side\":\"RIGHT\"},\"type\":\"ConnectorPlacement.EquallySpacedRectSide\",\"uuid\":\"0e6176f2-177c-4327-bcfa-9a190fe9083f\"},{\"content\":{\"connectorIds\":[\"LConn2\",\"In1\"],\"side\":\"TOP\"},\"type\":\"ConnectorPlacement.EquallySpacedRectSide\",\"uuid\":\"16faf74c-4635-4009-a5b3-33dd03b625c6\"},{\"content\":{\"connectorIds\":[\"RConn2\"],\"side\":\"BOTTOM\"},\"type\":\"ConnectorPlacement.EquallySpacedRectSide\",\"uuid\":\"2081d73b-bb08-4ad9-b5c8-e48a4e9c4e20\"}]},\"type\":\"ConnectorPlacement.EquallySpacedConnector\",\"uuid\":\"243e4075-206b-4747-a8bc-b8f10d9a577f\"}],\"packageUris\":[\"http://schema.mathworks.com/mf0/Connector/R2020b\"],\"version\":\"1.0\"}"
  Conductive Heat Transfer1 : fl_lib/Thermal/Thermal Elements/Conductive Heat Transfer  area=CoreVolume/CoreLength*(1-FuelFraction) m^2  thickness=0.5*CoreLength/N_nodes m  th_cond=k_graphite W/(m*K)  T_specify=off  T_priority=None  T=0 K  T_nominal_specify=off  T_nominal_unit=K  T_nominal_value=1  Q_specify=off  Q_priority=None  Q=0 W  Q_nominal_specify=off  Q_nominal_unit=W  Q_nominal_value=1
  Conductive Heat Transfer2 : fl_lib/Thermal/Thermal Elements/Conductive Heat Transfer  area=CoreVolume/CoreLength*(1-FuelFraction) m^2  thickness=0.5*CoreLength/N_nodes m  th_cond=k_graphite W/(m*K)  T_specify=off  T_priority=None  T=0 K  T_nominal_specify=off  T_nominal_unit=K  T_nominal_value=1  Q_specify=off  Q_priority=None  Q=0 W  Q_nominal_specify=off  Q_nominal_unit=W  Q_nominal_value=1
  Conductive Heat Transfer3 : fl_lib/Thermal/Thermal Elements/Conductive Heat Transfer  area=FuelGraphiteArea/N_nodes m^2  thickness=0.5*UnitCellGraphiteThickness m  th_cond=k_graphite W/(m*K)  T_specify=off  T_priority=None  T=0 K  T_nominal_specify=off  T_nominal_unit=K  T_nominal_value=1  Q_specify=off  Q_priority=None  Q=0 W  Q_nominal_specify=off  Q_nominal_unit=W  Q_nominal_value=1
  Constant Volume Chamber (TL) : fl_lib/Thermal Liquid/Elements/Constant Volume Chamber (TL)  volume=0.001 m^3  num_ports=foundation.enum.num_ports.two  area_A=0.01 m^2  area_B=0.01 m^2  area_C=0.01 m^2  area_D=0.01 m^2  p_I_specify=on  p_I_priority=None  p_I=P0 Pa  p_I_nominal_specify=off  p_I_nominal_unit=MPa  p_I_nominal_value=1  T_I_specify=on  T_I_priority=None  T_I=T0 K  T_I_nominal_specify=off  T_I_nominal_unit=K  T_I_nominal_value=1  u_chamber_specify=on  u_chamber_priority=None  u_chamber=cpMSRE J/kg  u_chamber_nominal_specify=off  u_chamber_nominal_unit=kJ/kg  u_chamber_nominal_value=1  rho_specify=on  rho_priority=None  rho=nominalFuelDensity kg/m^3  rho_nominal_specify=off  rho_nominal_unit=kg/m^3  rho_nominal_value=1
      settings: SourceProductBaseCode=SS  LogSimulationData=on  InternalSimscapePortConfiguration="{\"Bottom\":[],\"Left\":[{\"id\":\"A\",\"label\":\"A\",\"type\":\"foundation.thermal_liquid.thermal_liquid\"},{\"id\":\"H\",\"label\":\"H\",\"type\":\"foundation.thermal.thermal\"}],\"Right\":[{\"id\":\"B\",\"label\":\"B\",\"type\":\"foundation.thermal_liquid.thermal_liquid\"}],\"Top\":[]}"
  Controlled Heat Flow Rate Source : fl_lib/Thermal/Thermal Sources/Controlled Heat Flow Rate Source
      settings: LogSimulationData=on
  Convective Heat Transfer : fl_lib/Thermal/Thermal Elements/Convective Heat Transfer  area=fuelGraphiteArea/N_nodes m^2  heat_tr_coeff=fuelGraphiteHeatTransferCoefficient W/(m^2*K)  T_specify=off  T_priority=None  T=0 K  T_nominal_specify=off  T_nominal_unit=K  T_nominal_value=1  Q_specify=off  Q_priority=None  Q=0 W  Q_nominal_specify=off  Q_nominal_unit=W  Q_nominal_value=1
  Fuel Deposited : fl_lib/Physical Signals/Functions/PS Gain  gain=FuelDepositRatio*CoreVolume/N_nodes m^3
  Grahite Deposited : fl_lib/Thermal/Thermal Sources/Controlled Heat Flow Rate Source
      settings: LogSimulationData=on
  Graphite Deposited : fl_lib/Physical Signals/Functions/PS Gain  gain=(1-FuelDepositRatio)*CoreVolume/N_nodes m^3
  Pipe (TL) : SimscapeFluids_lib/Thermal Liquid/Pipes & Fittings/Pipe (TL)  dynamic_compressibility=simscape.enum.onoff.on  inertia=simscape.enum.onoff.off  num_segments=1  pipe_length=fuelChannelLength/N_nodes m  area=coreFlowArea m^2  Dh=0.1128 m  wall_spec=fluids.thermal_liquid.pipes_fittings.enum.wall_spec.rigid  Dh_rigid=fuelChannelHydrualicDiameter m  wall_compliance=1.2e-6 m/MPa  wall_time_constant=0.01 s  elevation_spec=foundation.enum.constant_variable.constant  elevation_gain=fuelChannelLength/N_nodes m  g=9.82 m/s^2  pressure_loss_spec=fluids.thermal_liquid.pipes_fittings.enum.PressureLossSpec.Haaland  length_add=1 m  roughness=surfaceRoughness m  Re_friction_TLU=[400, 1000, 1500, 3000, 4000, 6000, 10000, 20000, 40000, 60000, 100000, 100000000]  friction_factor_TLU=[.264, .112, .071, .0417, .0387, .0268, .025, .0232, .0226, .022, .0214, .0214]  shape_factor=64  Re_lam=2000  Re_tur=4000  mdot_nominal=[.1, 1] kg/s  p_diff_nominal=[.001, .01] MPa  mdot_threshold=1e-6 kg/s  heat_transfer_spec=fluids.thermal_liquid.pipes_fittings.enum.HeatTransferSpec.Gnielinski  mdot_nominal_heat=[0.1, 10000] kg/s  T_in_nominal=[T0, T0] K  T_out_nominal=[T0, T0] K  p_in_nominal_heat=[.101325, .101325] MPa  T_wall_nominal=[T0+1, T0+1] K  a_coeff=0.023  b_Re_power=0.8  c_Pr_power=0.4  Nu_lam=3.66  Re_Colburn_TLU=[100, 150, 1000]  Colburn_factor_TLU=[.019, .013, .002]  Re_Nu_TLU=[100, 150, 1000]  Pr_Nu_TLU=[1, 10]  Nu_TLU=[3.72, 4.21; 3.75, 4.44; 4.21, 7.15]  T0_vec=T0 K  p0_vec=P0+10000 Pa  mdot0=0.1 kg/s
      settings: SourceProductBaseCode=SH
  Temperature Sensor : fl_lib/Thermal/Thermal Sensors/Temperature Sensor
  Thermal Mass : fl_lib/Thermal/Thermal Elements/Thermal Mass  mass=CoreVolume*(1-FuelFraction)*rho_graphite/N_nodes kg  sp_heat=cp_graphite J/(K*kg)  T_specify=on  T_priority=High  T=T0 K  T_nominal_specify=off  T_nominal_unit=K  T_nominal_value=1  Q_specify=off  Q_priority=None  Q=0 W  Q_nominal_specify=off  Q_nominal_unit=W  Q_nominal_value=1
      settings: LogSimulationData=on
  Thermal Reference : fl_lib/Thermal/Thermal Elements/Thermal Reference
  Thermal Reference1 : fl_lib/Thermal/Thermal Elements/Thermal Reference
  Thermal Reference2 : fl_lib/Thermal/Thermal Elements/Thermal Reference
  Inlet : PMIOPort  Side=Left
  GraphiteA : PMIOPort  Port=2  Side=Left
  PowerDensity : PMIOPort  Port=3  Side=Left
  Outlet : PMIOPort  Port=4  Side=Right
  GraphiteB : PMIOPort  Port=5  Side=Right
  FuelTemp : PMIOPort  Port=6  Side=Right
  wires:
  GasRef/1 -> 2PModification/1
  connections:
  Grahite Deposited/LConn1 -- Conductive Heat Transfer3/RConn1 -- Conductive Heat Transfer2/RConn1 -- Thermal Mass/LConn1 -- Conductive Heat Transfer1/LConn1
  Graphite Deposited/LConn1 -- Fuel Deposited/LConn1 -- PowerDensity/RConn1
  Conductive Heat Transfer1/RConn1 -- GraphiteB/RConn1
  Grahite Deposited/RConn1 -- Graphite Deposited/RConn1
  GraphiteA/RConn1 -- Conductive Heat Transfer2/LConn1
  Controlled Heat Flow Rate Source/RConn2 -- Thermal Reference/LConn1
  Grahite Deposited/RConn2 -- Thermal Reference1/LConn1
  Fuel Deposited/RConn1 -- Controlled Heat Flow Rate Source/RConn1
  Outlet/RConn1 -- 2PModification/RConn1
  Temperature Sensor/RConn1 -- Thermal Reference2/LConn1
  Temperature Sensor/RConn2 -- FuelTemp/RConn1
  Inlet/RConn1 -- Constant Volume Chamber (TL)/LConn1
  Conductive Heat Transfer3/LConn1 -- Temperature Sensor/LConn1 -- Convective Heat Transfer/RConn1
  Constant Volume Chamber (TL)/LConn2 -- Convective Heat Transfer/LConn1 -- Controlled Heat Flow Rate Source/LConn1 -- Pipe (TL)/LConn2
  2PModification/RConn2 -- 2PModification/LConn1 -- Pipe (TL)/RConn1
  Constant Volume Chamber (TL)/RConn1 -- 2PModification/LConn2 -- Pipe (TL)/LConn1
